simulink model "Implementation"  (R2015a)
settings: Solver=ode3  StartTime=0.0  StopTime=50  RelTol=1e-3
values from neighbouring files (symbols this model uses):
  A = [3.3545 -4.3521 2.6058 -0.6082; 1 0 0 0; 0 1 0 0; 0 0 1 0]    [LQGm.m]    (also in Testes_planta.m = [3.11506910744011 -3.74010634305672 2.06382118501694 -0.4387)
  B = [1;0;0;0]    [LQGm.m]    (also in Testes_planta.m)
  C = [-0.0657 0.1152 0 0]    [LQGm.m]    (also in Testes_planta.m = [-0.0767099115028891 0.161398714293952 0 0])
  ExtensometerGain = -3.1481    [Testes_planta.m]
  Nbar = Nu+K*Nx    [LQGm.m]    (also in Testes_planta.m)
  PotentiometerGain = 180/5.3145    (= 33.8696020322)    [Testes_planta.m]
undefined symbols (not defined in the file or in its folder): K, M, MIO, National_Instruments, PCI
libraries: sldrtlib x2
settings Model: SimulationMode=external  ExtModeTrigDuration=20000  Creator=Alunos  LastModifiedBy=Alunos
settings HardwareCC: ProdIntDivRoundTo=Zero  ProdEndianess=LittleEndian  ProdHWDeviceType=Intel->x86/Pentium  TargetIntDivRoundTo=Zero  TargetEndianess=LittleEndian  TargetHWDeviceType=Intel->x86/Pentium
settings RTWCC: SystemTargetFile=rtwin.tlc  TemplateMakefile=rtwin.tmf  Description=Simulink Desktop Real-Time  RTWCompilerOptimization=on
settings CodeAppCC: MaxIdLength=95
settings RTWinTargetCC: TargetPreCompLibLocation=C:\Program Files\MATLAB\R2015a\toolbox\sldrt\lib\win32

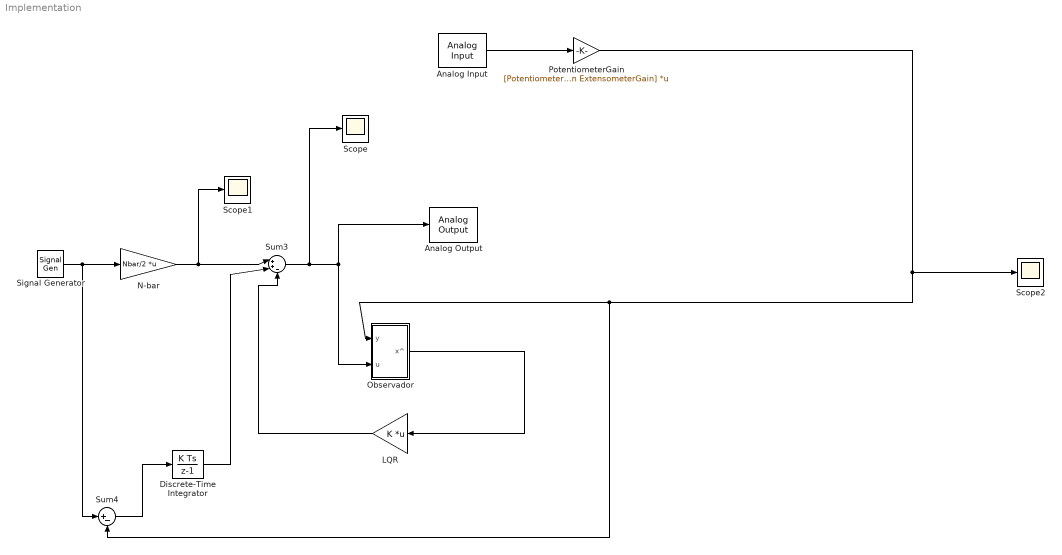
== system Implementation ==
  Analog Input : sldrtlib/Analog Input  SampleTime=0.02  MaxMissedTicks=10  ShowMissedTicks=off  YieldWhenWaiting=off  DrvName=National_Instruments/PCI-MIO-16E-4  DrvAddress=4294967295  DrvOptions=[0 0 0 0 0 0]  Channels=[1 2]  RangeMode=1  VoltRange=1  DataType=1
      settings: AttributesFormatString=National Instruments\nPCI-MIO-16E-4 [auto]
  Analog Output : sldrtlib/Analog Output  SampleTime=0.02  MaxMissedTicks=10  ShowMissedTicks=off  YieldWhenWaiting=off  DrvName=National_Instruments/PCI-MIO-16E-4  DrvAddress=4294967295  DrvOptions=[0 0 0 0 0 0]  Channels=1  RangeMode=1  VoltRange=1  InitialValue=0  FinalValue=0
      settings: AttributesFormatString=National Instruments\nPCI-MIO-16E-4 [auto]
  Discrete-Time Integrator : DiscreteIntegrator  gainval=1e-2  InitialConditionSetting=State (most efficient)
  LQR : Gain  Gain=K  Multiplication=Matrix(K*u)
  N-bar : Gain  Gain=Nbar/2  Multiplication=Matrix(K*u)
  Observador : Subsystem
  PotentiometerGain : Gain  Gain=[PotentiometerGain ExtensometerGain]  Multiplication=Matrix(K*u)
  Scope : Scope
  Scope1 : Scope
  Scope2 : Scope
      settings: SaveName=TestData
  Signal Generator : SignalGenerator  WaveForm=square  Amplitude=30  Frequency=0.2
  Sum3 : Sum  Inputs=|++-
  Sum4 : Sum  Inputs=|+-
  wires:
  Signal Generator/1 -> Sum4/1, N-bar/1
  LQR/1 -> Sum3/3
  PotentiometerGain/1 -> Observador/1(y), Sum4/2, Scope2/1
  Observador/1(x^) -> LQR/1
  N-bar/1 -> Sum3/1, Scope1/1
  Sum3/1 -> Scope/1, Analog Output/1, Observador/2(u)
  Sum4/1 -> Discrete-Time Integrator/1
  Discrete-Time Integrator/1 -> Sum3/2
  Analog Input/1 -> PotentiometerGain/1

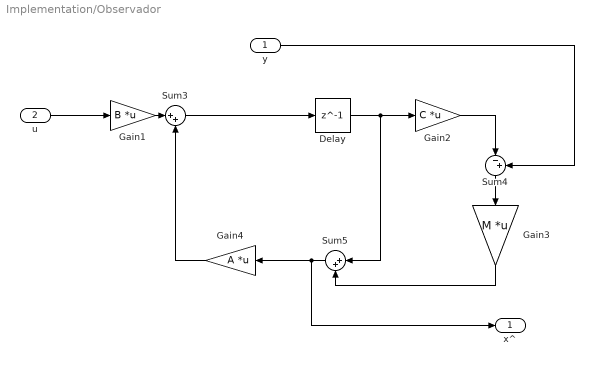
== system Implementation/Observador ==
  y : Inport
  u : Inport  Port=2
  Delay : Delay  DelayLength=1  InitialCondition=0
  Gain1 : Gain  Gain=B  Multiplication=Matrix(K*u)
  Gain2 : Gain  Gain=C  Multiplication=Matrix(K*u)
  Gain3 : Gain  Gain=M  Multiplication=Matrix(K*u)
  Gain4 : Gain  Gain=A  Multiplication=Matrix(K*u)
  Sum3 : Sum  Inputs=|++
  Sum4 : Sum  Inputs=|-+
  Sum5 : Sum  Inputs=|++
  x^ : Outport
  wires:
  u/1 -> Gain1/1
  Gain1/1 -> Sum3/1
  Sum4/1 -> Gain3/1
  Gain3/1 -> Sum5/2
  Gain4/1 -> Sum3/2
  Sum5/1 -> x^/1, Gain4/1
  Delay/1 -> Sum5/1, Gain2/1
  Gain2/1 -> Sum4/1
  Sum3/1 -> Delay/1
  y/1 -> Sum4/2
